simulink model "SUBS_CABLE_CARRO"  (R2024b)
settings: Solver=VariableStepAuto  StartTime=0.0  StopTime=10.0  RelTol=1e-3
undefined symbols (not defined in the file): btw, Ktw
settings Model: Creator=juani  LastModifiedBy=juani

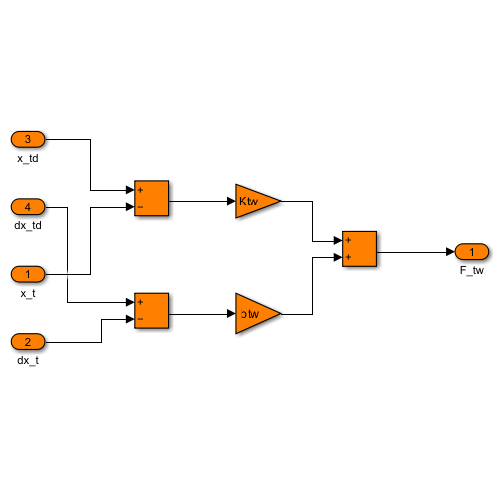
[thumbnail: Simulink's stored preview of the top-level diagram]
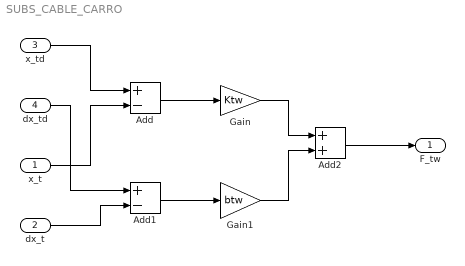
== system SUBS_CABLE_CARRO ==
  x_t : Inport
  dx_t : Inport  Port=2
  x_td : Inport  Port=3
  dx_td : Inport  Port=4
  Add : Sum  Inputs=+-
  Add1 : Sum  Inputs=+-
  Add2 : Sum
  Gain : Gain  Gain=Ktw
  Gain1 : Gain  Gain=btw
  F_tw : Outport
  wires:
  x_td/1 -> Add/1
  x_t/1 -> Add/2
  dx_td/1 -> Add1/1
  dx_t/1 -> Add1/2
  Add/1 -> Gain/1
  Add1/1 -> Gain1/1
  Gain/1 -> Add2/1
  Gain1/1 -> Add2/2
  Add2/1 -> F_tw/1
